simulink model "MSDR_DH_DeplV1sim"  (R2019a)
settings: Solver=ode45  StartTime=0.0  StopTime=simtime  FixedStep=0.1  MaxStep=ts_max  RelTol=rel_tolerance
values from neighbouring files (symbols this model uses):
  a_f = 1E-5*depl_fuel_temp_coef(depl_index)    [MSDR_DH_DeplV1para.m]
  a_g = 1E-5*depl_grap_temp_coef(depl_index)    [MSDR_DH_DeplV1para.m]
  A_s = 1.2245    [MSDR_DH_DeplV1para.m]
  beta = depl_beta(depl_index,:)    [MSDR_DH_DeplV1para.m]
  beta_t = sum(beta)    [MSDR_DH_DeplV1para.m]
  Cp_f = depl_Cp_Fuel_coef*1.355616e-3    [MSDR_DH_DeplV1para.m]
  Cp_p = Cp_s_shx    [MSDR_DH_DeplV1para.m]
  Cp_s = Cp_s*1e-6    (= 3.588208e-09)    [MSDR_DH_DeplV1para.m]
  Cp_sc = 4761.392e-6    (= 0.004761392)    [MSDR_DH_DeplV1para.m]
  Cp_w = 456.056e-6    (= 0.000456056)    [MSDR_DH_DeplV1para.m]
  D_it = 0.0141478    [MSDR_DH_DeplV1para.m]
  D_ot = 0.015875    [MSDR_DH_DeplV1para.m]
  DHRS_TIME_K = 10    [MSDR_DH_DeplV1para.m]
  dHs_dPs = -0.042433622114357    (= -0.0424336221144)    [MSDR_DH_DeplV1para.m]
  Epsilon = 1E-3    (= 0.001)    [MSDR_DH_DeplV1para.m]
  Fiss_factor = 2.464783802008740e-03    (= 0.00246478380201)    [MSDR_DH_DeplV1para.m]
  gamma0 = 9.635981959409105e-01    (= 0.963598195941)    [MSDR_DH_DeplV1para.m]
  gamma1 = 3.560674858154914e-02    (= 0.0356067485815)    [MSDR_DH_DeplV1para.m]
  gamma2 = 7.950554775404400e-04    (= 0.00079505547754)    [MSDR_DH_DeplV1para.m]
  gamma_I = 5.1135e-2    (= 0.051135)    [MSDR_DH_DeplV1para.m]
  gamma_Pm = 1.08E-2    (= 0.0108)    [MSDR_DH_DeplV1para.m]
  gamma_Xe = 1.1628e-2    (= 0.011628)    [MSDR_DH_DeplV1para.m]
  h_pw = h_s_shx    [MSDR_DH_DeplV1para.m]
  h_wb = 13349.334646671E-6    (= 0.0133493346467)    [MSDR_DH_DeplV1para.m]
  h_ws = 5732.378387768E-6    (= 0.00573237838777)    [MSDR_DH_DeplV1para.m]
  h_wsc = 8385.005556375E-6    (= 0.00838500555638)    [MSDR_DH_DeplV1para.m]
  hA_fg = [h_fg*A_fg/2, h_fg*A_fg/2]    [MSDR_DH_DeplV1para.m]
  hA_p_phx1 = h_p_phx*A_p_phx    [MSDR_DH_DeplV1para.m]
  hA_p_phx2 = h_p_phx*A_p_phx    [MSDR_DH_DeplV1para.m]
  hA_p_phx3 = h_p_phx*A_p_phx    [MSDR_DH_DeplV1para.m]
  hA_p_phx4 = h_p_phx*A_p_phx    [MSDR_DH_DeplV1para.m]
  hA_p_phx5 = h_p_phx*A_p_phx    [MSDR_DH_DeplV1para.m]
  hA_p_phx6 = h_p_phx*A_p_phx    [MSDR_DH_DeplV1para.m]
  hA_p_shx1 = h_p_shx*A_p_shx    [MSDR_DH_DeplV1para.m]
  hA_p_shx2 = h_p_shx*A_p_shx    [MSDR_DH_DeplV1para.m]
  hA_p_shx3 = h_p_shx*A_p_shx    [MSDR_DH_DeplV1para.m]
  hA_p_shx4 = h_p_shx*A_p_shx    [MSDR_DH_DeplV1para.m]
  hA_p_shx5 = h_p_shx*A_p_shx    [MSDR_DH_DeplV1para.m]
  hA_p_shx6 = h_p_shx*A_p_shx    [MSDR_DH_DeplV1para.m]
  hA_s_phx1 = h_s_phx*A_s_phx    [MSDR_DH_DeplV1para.m]
  hA_s_phx2 = h_s_phx*A_s_phx    [MSDR_DH_DeplV1para.m]
  hA_s_phx3 = h_s_phx*A_s_phx    [MSDR_DH_DeplV1para.m]
  hA_s_phx4 = h_s_phx*A_s_phx    [MSDR_DH_DeplV1para.m]
  hA_s_phx5 = h_s_phx*A_s_phx    [MSDR_DH_DeplV1para.m]
  hA_s_phx6 = h_s_phx*A_s_phx    [MSDR_DH_DeplV1para.m]
  hA_s_shx1 = h_s_shx*A_s_shx    [MSDR_DH_DeplV1para.m]
  hA_s_shx2 = h_s_shx*A_s_shx    [MSDR_DH_DeplV1para.m]
  hA_s_shx3 = h_s_shx*A_s_shx    [MSDR_DH_DeplV1para.m]
  hA_s_shx4 = h_s_shx*A_s_shx    [MSDR_DH_DeplV1para.m]
  hA_s_shx5 = h_s_shx*A_s_shx    [MSDR_DH_DeplV1para.m]
  hA_s_shx6 = h_s_shx*A_s_shx    [MSDR_DH_DeplV1para.m]
  I_0 = gamma_I*Sig_f_msdr*phi_0/lam_I    [MSDR_DH_DeplV1para.m]
  Ifa = [0.25, 0.25]    [MSDR_DH_DeplV1para.m]
  Ifb = [0.25, 0.25]    [MSDR_DH_DeplV1para.m]
  Ig = [0.5, 0.5]    [MSDR_DH_DeplV1para.m]
  K_1 = 11.632248097704855    (= 11.6322480977)    [MSDR_DH_DeplV1para.m]
  K_4 = b(1)    [MSDR_DH_DeplV1para.m]
  K_5 = a(1)    [MSDR_DH_DeplV1para.m]
  K_b = 12.834854076292217    (= 12.8348540763)    [MSDR_DH_DeplV1para.m]
  K_pump = 1/5    (= 0.2)    [MSDR_DH_DeplV1para.m]
  K_sc = -17.615718797133468    (= -17.6157187971)    [MSDR_DH_DeplV1para.m]
  ka = [0.235, 0.235]    [MSDR_DH_DeplV1para.m]
  kb = [0.235, 0.235]    [MSDR_DH_DeplV1para.m]
  kga = [0.015, 0.015]    [MSDR_DH_DeplV1para.m]
  kgb = [0.015, 0.015]    [MSDR_DH_DeplV1para.m]
  L = 8.5344    [MSDR_DH_DeplV1para.m]
  L_b = 2.3645    [MSDR_DH_DeplV1para.m]
  L_s = 4.723    [MSDR_DH_DeplV1para.m]
  Lam = depl_Lam(depl_index)    [MSDR_DH_DeplV1para.m]
  lam = [1.240E-02, 3.05E-02, 1.11E-01, 3.01E-01, 1.140E+00, 3.014E+00]    [MSDR_DH_DeplV1para.m]
  lam_bubl = 2.0e-2    (= 0.02)    [MSDR_DH_DeplV1para.m]
  lam_I = 2.875e-5    (= 2.875e-05)    [MSDR_DH_DeplV1para.m]
  lam_Pm = log(2)/(2.21*24*3600)    [MSDR_DH_DeplV1para.m]
  lam_Xe = 2.0916e-5    (= 2.0916e-05)    [MSDR_DH_DeplV1para.m]
  lambda0 = 0.0945298    [MSDR_DH_DeplV1para.m]
  lambda1 = 0.00441957    [MSDR_DH_DeplV1para.m]
  lambda2 = 8.60979e-05    [MSDR_DH_DeplV1para.m]
  m_3m = W_3*2    (= 8618.207327)    [MSDR_DH_DeplV1para.m]
  m_f_t = total_mp_phx + core_fm + mp_phxm*3 + m_fm    [MSDR_DH_DeplV1para.m]
  m_fm = W_f*1    (= 4989.48)    [MSDR_DH_DeplV1para.m]
  M_stm = 0.018    [MSDR_DH_DeplV1para.m]
  mcp_fa = mfa*Cp_f    [MSDR_DH_DeplV1para.m]
  mcp_fb = mfb*Cp_f    [MSDR_DH_DeplV1para.m]
  mcp_g = mg*Cp_g    [MSDR_DH_DeplV1para.m]
  mcp_p_phx1 = Cp_p_phx*mp_phx1    [MSDR_DH_DeplV1para.m]
  mcp_p_phx2 = Cp_p_phx*mp_phx2    [MSDR_DH_DeplV1para.m]
  mcp_p_phx3 = Cp_p_phx*mp_phx3    [MSDR_DH_DeplV1para.m]
  mcp_p_phx4 = Cp_p_phx*mp_phx4    [MSDR_DH_DeplV1para.m]
  mcp_p_phx5 = Cp_p_phx*mp_phx5    [MSDR_DH_DeplV1para.m]
  mcp_p_phx6 = Cp_p_phx*mp_phx6    [MSDR_DH_DeplV1para.m]
  mcp_p_shx1 = Cp_p_shx*mp_shx1    [MSDR_DH_DeplV1para.m]
  mcp_p_shx2 = Cp_p_shx*mp_shx2    [MSDR_DH_DeplV1para.m]
  mcp_p_shx3 = Cp_p_shx*mp_shx3    [MSDR_DH_DeplV1para.m]
  mcp_p_shx4 = Cp_p_shx*mp_shx4    [MSDR_DH_DeplV1para.m]
  mcp_p_shx5 = Cp_p_shx*mp_shx5    [MSDR_DH_DeplV1para.m]
  mcp_p_shx6 = Cp_p_shx*mp_shx6    [MSDR_DH_DeplV1para.m]
  mcp_s_phx1 = Cp_s_phx*ms_phx1    [MSDR_DH_DeplV1para.m]
  mcp_s_phx2 = Cp_s_phx*ms_phx2    [MSDR_DH_DeplV1para.m]
  mcp_s_phx3 = Cp_s_phx*ms_phx3    [MSDR_DH_DeplV1para.m]
  mcp_s_phx4 = Cp_s_phx*ms_phx4    [MSDR_DH_DeplV1para.m]
  mcp_s_phx5 = Cp_s_phx*ms_phx5    [MSDR_DH_DeplV1para.m]
  mcp_s_phx6 = Cp_s_phx*ms_phx6    [MSDR_DH_DeplV1para.m]
  mcp_s_shx1 = Cp_s_shx*ms_shx1    [MSDR_DH_DeplV1para.m]
  mcp_s_shx2 = Cp_s_shx*ms_shx1    [MSDR_DH_DeplV1para.m]
  mcp_s_shx3 = Cp_s_shx*ms_shx1    [MSDR_DH_DeplV1para.m]
  mcp_s_shx4 = Cp_s_shx*ms_shx1    [MSDR_DH_DeplV1para.m]
  mcp_s_shx5 = Cp_s_shx*ms_shx1    [MSDR_DH_DeplV1para.m]
  mcp_s_shx6 = Cp_s_shx*ms_shx1    [MSDR_DH_DeplV1para.m]
  mcp_t_phx1 = Cp_t_phx*mt_phx1    [MSDR_DH_DeplV1para.m]
  mcp_t_phx2 = Cp_t_phx*mt_phx2    [MSDR_DH_DeplV1para.m]
  mcp_t_phx3 = Cp_t_phx*mt_phx3    [MSDR_DH_DeplV1para.m]
  mcp_t_phx4 = Cp_t_phx*mt_phx4    [MSDR_DH_DeplV1para.m]
  mcp_t_phx5 = Cp_t_phx*mt_phx5    [MSDR_DH_DeplV1para.m]
  mcp_t_phx6 = Cp_t_phx*mt_phx6    [MSDR_DH_DeplV1para.m]
  mcp_t_shx1 = Cp_t_phx*mt_shx1    [MSDR_DH_DeplV1para.m]
  mcp_t_shx2 = Cp_t_phx*mt_shx2    [MSDR_DH_DeplV1para.m]
  mcp_t_shx3 = Cp_t_phx*mt_shx3    [MSDR_DH_DeplV1para.m]
  mcp_t_shx4 = Cp_t_phx*mt_shx4    [MSDR_DH_DeplV1para.m]
  mcp_t_shx5 = Cp_t_phx*mt_shx5    [MSDR_DH_DeplV1para.m]
  mcp_t_shx6 = Cp_t_phx*mt_shx6    [MSDR_DH_DeplV1para.m]
  ... (+159 more)
undefined symbols (not defined in the file or in its folder): C0, DHRS_MODE, DHRS_Power, DHRS_time, ln, P, Trip_P1_pump, Trip_P2_pump, Trip_P3_pump, Trip_S1_pump, Trip_S2_pump, Trip_S3_pump, Trip_T1_pump, Trip_T2_pump, Trip_T3_pump, Trip_UHX
libraries: simulink x2
(part 2 of 4)

== system MSDR_DH_DeplV1sim/SECONDARY SIDE/OTSG + BALANCE OF PLANT ==
  HITEC_INLET : Inport
  POWER LEVEL : Inport  Port=2
  HITEC_FLOW_FRAC : Inport  Port=3
  HITEC_HTC_FRAC : Inport  Port=4
  Clock : Clock
  Clock1 : Clock
  Constant1 : Constant  Value=0
  Constant12 : Constant  Value=T_fw
  Constant13 : Constant  Value=W_p0
  Constant2 : Constant
  Constant4 : Constant  Value=12.5
  Display{12,14..15,47} (4 alike) : Display
  ONCE-THROUGH STEAM GENERATOR : Subsystem
  Product : Product
  SHX TO PHX DELAY1 : VariableTransportDelay  MaximumDelay=1000000000000  InitialOutput=T0_s_shx5(4)
  Switch : Switch  Criteria=u2 > Threshold  Threshold=Trip_UHX
  Switch1 : Switch  Threshold=Trip_UHX
  VAR DELAY FUNC3 : Fcn  Expr=tau_ostg_shx/u
  HITEC_OUTLET : Outport
  wires:
  ONCE-THROUGH STEAM GENERATOR/4(STEAM FLOW RATE) -> [steam_flow_OTSG], Display15/1
  ONCE-THROUGH STEAM GENERATOR/2(HITEC OUTLET TEMPERATURE) -> Display47/1, Switch/3
  ONCE-THROUGH STEAM GENERATOR/1(STEAM TEMPERATURE) -> Display12/1, [T_steam_OTSG]
  ONCE-THROUGH STEAM GENERATOR/3(STEAM PRESSURE) -> [P_steam_OTSG], Display14/1
  HITEC_INLET/1 -> ONCE-THROUGH STEAM GENERATOR/1(HITEC INLET TEMPERATURE), [HITEC_IN_TEMP]
  Constant4/1 -> ONCE-THROUGH STEAM GENERATOR/6(PRESSURE SET POINT)
  Constant12/1 -> ONCE-THROUGH STEAM GENERATOR/2(FEEDWATER INLET TEMPERATURE)
  HITEC_HTC_FRAC/1 -> ONCE-THROUGH STEAM GENERATOR/4(HITEC HEAT TRANSFER FRAC)
  Constant13/1 -> Product/2
  HITEC_FLOW_FRAC/1 -> Product/1, [HITEC_FLOW_FRAC]
  Product/1 -> ONCE-THROUGH STEAM GENERATOR/3(HITEC FLOW RATE)
  Switch/1 -> HITEC_OUTLET/1
  Clock/1 -> Switch/2
  [HITEC_FLOW_FRAC] -> VAR DELAY FUNC3/1
  [HITEC_IN_TEMP] -> SHX TO PHX DELAY1/1
  VAR DELAY FUNC3/1 -> SHX TO PHX DELAY1/2
  SHX TO PHX DELAY1/1 -> Switch/1
  Clock1/1 -> Switch1/2
  Constant1/1 -> Switch1/1
  POWER LEVEL/1 -> ONCE-THROUGH STEAM GENERATOR/5(POWER)
  Switch1/1 -> ONCE-THROUGH STEAM GENERATOR/Enable
  Constant2/1 -> Switch1/3

== system MSDR_DH_DeplV1sim/SECONDARY SIDE/Variant Subsystem ==
  HITEC_INLET : Inport
  POWER LEVEL : Inport  Port=2
  HITEC_FLOW_FRAC : Inport  Port=3
  HITEC_HTC_FRAC : Inport  Port=4
  OTSG : Subsystem  VariantControl=OTSG
  UHX : Subsystem  VariantControl=UHX
  HITEC_OUTLET : Outport

== system MSDR_DH_DeplV1sim/HEAT EXCHANGERS/HEAT EXCHANGER LOOP 1/PHX PRIM MIXING ==
  Tp_phx1 : Inport
  Tp_phx2 : Inport  Port=2
  p_flow_frac : Inport  Port=3
  Decay Heat : Inport  Port=4
  Fcn : Fcn  Expr=u[3]*Wp_phx1/mp_phxm*(u[1]-u[4]) + u[3]*Wp_phx2/mp_phxm*(u[2]-u[4]) + u(5)*P*mp_phxm/(m_f_t*mp_phxm*Cp_f)
  Integrator : Integrator  InitialCondition=Tf_in
  Mux : Mux  Inputs=5
  Tp_phx_mix : Outport
  wires:
  Tp_phx1/1 -> Mux/1
  Tp_phx2/1 -> Mux/2
  Mux/1 -> Fcn/1
  p_flow_frac/1 -> Mux/3
  Fcn/1 -> Integrator/1
  Integrator/1 -> Mux/4, Tp_phx_mix/1
  Decay Heat/1 -> Mux/5

== system MSDR_DH_DeplV1sim/HEAT EXCHANGERS/HEAT EXCHANGER LOOP 1/PHX SEC MIXING ==
  Ts_phx1 : Inport
  Ts_phx2 : Inport  Port=2
  s_flow_frac : Inport  Port=3
  Fcn : Fcn  Expr=u[3]*Ws_phx1/ms_phxm*(u[1]-u[4]) + u[3]*Ws_phx2/ms_phxm*(u[2]-u[4])
  Integrator : Integrator  InitialCondition=T0_s_phx1(4)
  Mux : Mux
  Ts_phx_mix : Outport
  wires:
  Ts_phx1/1 -> Mux/1
  Ts_phx2/1 -> Mux/2
  Mux/1 -> Fcn/1
  s_flow_frac/1 -> Mux/3
  Fcn/1 -> Integrator/1
  Integrator/1 -> Ts_phx_mix/1, Mux/4

== system MSDR_DH_DeplV1sim/HEAT EXCHANGERS/HEAT EXCHANGER LOOP 1/PHX//SHX PUMP ==
  Clock1 : Clock
  Fcn1 : Fcn  Expr=(1-therm_conv)*exp(-K_pump*(u))+therm_conv
  H.T.C. as f(flow_fraction) : Fcn  Expr=0.8215*u^6-4.108*u^5+7.848*u^4-7.165*u^3+3.004*u^2+0.5903*u+0.008537
  Pump Trip Time : TransportDelay  DelayTime=Trip_S1_pump  BufferSize=4096
  FLOW FRACTION : Outport
  HEAT TRANSFER FRACTION : Outport  Port=2
  wires:
  H.T.C. as f(flow_fraction)/1 -> HEAT TRANSFER FRACTION/1
  Clock1/1 -> Pump Trip Time/1
  Pump Trip Time/1 -> Fcn1/1
  Fcn1/1 -> FLOW FRACTION/1, H.T.C. as f(flow_fraction)/1

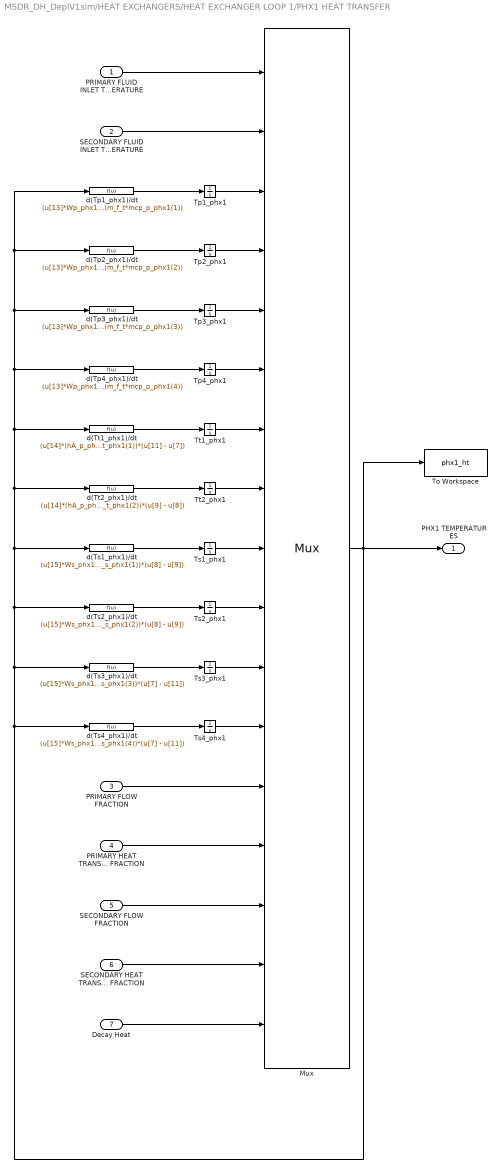
== system MSDR_DH_DeplV1sim/HEAT EXCHANGERS/HEAT EXCHANGER LOOP 1/PHX1 HEAT TRANSFER ==
  PRIMARY FLUID INLET TEMPERATURE : Inport
  SECONDARY FLUID INLET TEMPERATURE : Inport  Port=2
  PRIMARY FLOW FRACTION : Inport  Port=3
  PRIMARY HEAT TRANSFER FRACTION : Inport  Port=4
  SECONDARY FLOW FRACTION : Inport  Port=5
  SECONDARY HEAT TRANSFER FRACTION : Inport  Port=6
  Decay Heat : Inport  Port=7
  Mux : Mux  Inputs=17
      settings: DisplayOption=signals
  To Workspace : ToWorkspace  VariableName=phx1_ht  SampleTime=-1
  Tp1_phx1 : Integrator  InitialCondition=T0_p_phx1(1)
  Tp2_phx1 : Integrator  InitialCondition=T0_p_phx1(2)
  "Tp3_phx1 " : Integrator  InitialCondition=T0_p_phx1(3)
  Tp4_phx1 : Integrator  InitialCondition=T0_p_phx1(4)
  Ts1_phx1 : Integrator  InitialCondition=T0_s_phx1(1)
  Ts2_phx1 : Integrator  InitialCondition=T0_s_phx1(2)
  Ts3_phx1 : Integrator  InitialCondition=T0_s_phx1(3)
  Ts4_phx1 : Integrator  InitialCondition=T0_s_phx1(4)
  Tt1_phx1 : Integrator  InitialCondition=T0_t_phx1(1)
  Tt2_phx1 : Integrator  InitialCondition=T0_t_phx1(2)
  d(Tp1_phx1)/dt : Fcn  Expr=(u[13]*Wp_phx1/mp_phx1(1))*(u[1] - u[3]) + (u[14]*hA_p_phx1(1)/mcp_p_phx1(1))*(u[7] - u[3]) + u(17)*P*mp_phx1(1)/(m_f_t*mcp_p_phx1(1))
  d(Tp2_phx1)/dt : Fcn  Expr=(u[13]*Wp_phx1/mp_phx1(2))*(u[3] - u[4]) + (u[14]*hA_p_phx1(2)/mcp_p_phx1(2))*(u[7] - u[3]) + u(17)*P*mp_phx1(2)/(m_f_t*mcp_p_phx1(2))
  d(Tp3_phx1)/dt : Fcn  Expr=(u[13]*Wp_phx1/mp_phx1(3))*(u[4] - u[5]) + (u[14]*hA_p_phx1(3)/mcp_p_phx1(3))*(u[8] - u[5]) + u(17)*P*mp_phx1(3)/(m_f_t*mcp_p_phx1(3))
  d(Tp4_phx1)/dt : Fcn  Expr=(u[13]*Wp_phx1/mp_phx1(4))*(u[5] - u[6]) + (u[14]*hA_p_phx1(4)/mcp_p_phx1(4))*(u[8] - u[5]) + u(17)*P*mp_phx1(4)/(m_f_t*mcp_p_phx1(4))
  d(Ts1_phx1)/dt : Fcn  Expr=(u[15]*Ws_phx1/ms_phx1(1))*(u[2] - u[9]) + (u[16]*hA_s_phx1(1)/mcp_s_phx1(1))*(u[8] - u[9])
  d(Ts2_phx1)/dt : Fcn  Expr=(u[15]*Ws_phx1/ms_phx1(2))*(u[9] - u[10]) + (u[16]*hA_s_phx1(2)/mcp_s_phx1(2))*(u[8] - u[9])
  d(Ts3_phx1)/dt : Fcn  Expr=(u[15]*Ws_phx1/ms_phx1(3))*(u[10] - u[11]) + (u[16]*hA_s_phx1(3)/mcp_s_phx1(3))*(u[7] - u[11])
  d(Ts4_phx1)/dt : Fcn  Expr=(u[15]*Ws_phx1/ms_phx1(4))*(u[11] - u[12]) + (u[16]*hA_s_phx1(4)/mcp_s_phx1(4))*(u[7] - u[11])
  d(Tt1_phx1)/dt : Fcn  Expr=(u[14]*(hA_p_phx1(1) + hA_p_phx1(2))/mcp_t_phx1(1))*(u[3] - u[7]) + (u[16]*(hA_s_phx1(1) + hA_s_phx1(2))/mcp_t_phx1(1))*(u[11] - u[7])
  d(Tt2_phx1)/dt : Fcn  Expr=(u[14]*(hA_p_phx1(3) + hA_p_phx1(4))/mcp_t_phx1(2))*(u[5] - u[8]) + (u[16]*(hA_s_phx1(3) + hA_s_phx1(4))/mcp_t_phx1(2))*(u[9] - u[8])
  PHX1 TEMPERATURES : Outport
  wires:
  Ts1_phx1/1 -> Mux/9
  Ts2_phx1/1 -> Mux/10
  d(Ts2_phx1)/dt/1 -> Ts2_phx1/1
  d(Tp4_phx1)/dt/1 -> Tp4_phx1/1
  Tt1_phx1/1 -> Mux/7
  d(Tp2_phx1)/dt/1 -> Tp2_phx1/1
  Tp4_phx1/1 -> Mux/6
  d(Tt2_phx1)/dt/1 -> Tt2_phx1/1
  SECONDARY FLUID INLET TEMPERATURE/1 -> Mux/2
  Tt2_phx1/1 -> Mux/8
  Mux/1 -> To Workspace/1, PHX1 TEMPERATURES/1, d(Ts4_phx1)/dt/1, d(Ts3_phx1)/dt/1, d(Ts1_phx1)/dt/1, d(Tt2_phx1)/dt/1, d(Tt1_phx1)/dt/1, d(Tp4_phx1)/dt/1, d(Tp3_phx1)/dt/1, d(Tp2_phx1)/dt/1, d(Tp1_phx1)/dt/1, d(Ts2_phx1)/dt/1
  d(Tp1_phx1)/dt/1 -> Tp1_phx1/1
  d(Ts4_phx1)/dt/1 -> Ts4_phx1/1
  Tp1_phx1/1 -> Mux/3
  d(Ts1_phx1)/dt/1 -> Ts1_phx1/1
  d(Ts3_phx1)/dt/1 -> Ts3_phx1/1
  Ts3_phx1/1 -> Mux/11
  Ts4_phx1/1 -> Mux/12
  "Tp3_phx1 "/1 -> Mux/5
  d(Tp3_phx1)/dt/1 -> "Tp3_phx1 "/1
  Tp2_phx1/1 -> Mux/4
  d(Tt1_phx1)/dt/1 -> Tt1_phx1/1
  PRIMARY FLUID INLET TEMPERATURE/1 -> Mux/1
  PRIMARY FLOW FRACTION/1 -> Mux/13
  PRIMARY HEAT TRANSFER FRACTION/1 -> Mux/14
  SECONDARY HEAT TRANSFER FRACTION/1 -> Mux/16
  SECONDARY FLOW FRACTION/1 -> Mux/15
  Decay Heat/1 -> Mux/17

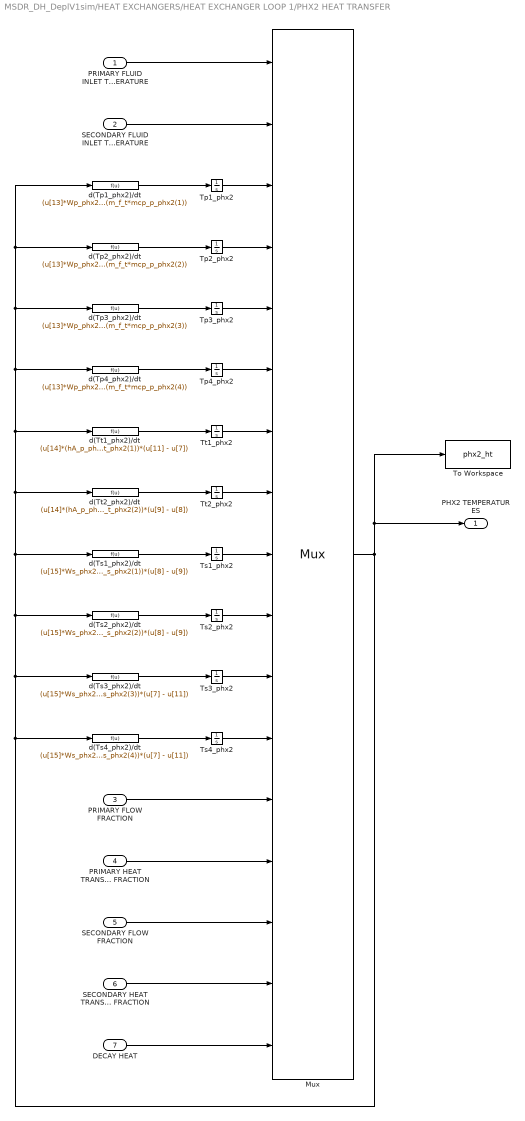
== system MSDR_DH_DeplV1sim/HEAT EXCHANGERS/HEAT EXCHANGER LOOP 1/PHX2 HEAT TRANSFER ==
  PRIMARY FLUID INLET TEMPERATURE : Inport
  SECONDARY FLUID INLET TEMPERATURE : Inport  Port=2
  PRIMARY FLOW FRACTION : Inport  Port=3
  PRIMARY HEAT TRANSFER FRACTION : Inport  Port=4
  SECONDARY FLOW FRACTION : Inport  Port=5
  SECONDARY HEAT TRANSFER FRACTION : Inport  Port=6
  DECAY HEAT : Inport  Port=7
  Mux : Mux  Inputs=17
      settings: DisplayOption=signals
  To Workspace : ToWorkspace  VariableName=phx2_ht  SampleTime=-1
  Tp1_phx2 : Integrator  InitialCondition=T0_p_phx2(1)
  Tp2_phx2 : Integrator  InitialCondition=T0_p_phx1(2)
  "Tp3_phx2 " : Integrator  InitialCondition=T0_p_phx2(3)
  Tp4_phx2 : Integrator  InitialCondition=T0_p_phx2(4)
  Ts1_phx2 : Integrator  InitialCondition=T0_s_phx2(1)
  Ts2_phx2 : Integrator  InitialCondition=T0_s_phx2(2)
  Ts3_phx2 : Integrator  InitialCondition=T0_s_phx2(3)
  Ts4_phx2 : Integrator  InitialCondition=T0_s_phx2(4)
  Tt1_phx2 : Integrator  InitialCondition=T0_t_phx2(1)
  Tt2_phx2 : Integrator  InitialCondition=T0_t_phx2(2)
  d(Tp1_phx2)/dt : Fcn  Expr=(u[13]*Wp_phx2/mp_phx2(1))*(u[1] - u[3]) + (u[14]*hA_p_phx2(1)/mcp_p_phx2(1))*(u[7] - u[3]) + u(17)*P*mp_phx2(1)/(m_f_t*mcp_p_phx2(1))
  d(Tp2_phx2)/dt : Fcn  Expr=(u[13]*Wp_phx2/mp_phx2(2))*(u[3] - u[4]) + (u[14]*hA_p_phx2(2)/mcp_p_phx2(2))*(u[7] - u[3]) + u(17)*P*mp_phx2(2)/(m_f_t*mcp_p_phx2(2))
  d(Tp3_phx2)/dt : Fcn  Expr=(u[13]*Wp_phx2/mp_phx2(3))*(u[4] - u[5]) + (u[14]*hA_p_phx2(3)/mcp_p_phx2(3))*(u[8] - u[5]) + u(17)*P*mp_phx2(3)/(m_f_t*mcp_p_phx2(3))
  d(Tp4_phx2)/dt : Fcn  Expr=(u[13]*Wp_phx2/mp_phx2(4))*(u[5] - u[6]) + (u[14]*hA_p_phx2(4)/mcp_p_phx2(4))*(u[8] - u[5]) + u(17)*P*mp_phx2(4)/(m_f_t*mcp_p_phx2(4))
  d(Ts1_phx2)/dt : Fcn  Expr=(u[15]*Ws_phx2/ms_phx2(1))*(u[2] - u[9]) + (u[16]*hA_s_phx2(1)/mcp_s_phx2(1))*(u[8] - u[9])
  d(Ts2_phx2)/dt : Fcn  Expr=(u[15]*Ws_phx2/ms_phx2(2))*(u[9] - u[10]) + (u[16]*hA_s_phx2(2)/mcp_s_phx2(2))*(u[8] - u[9])
  d(Ts3_phx2)/dt : Fcn  Expr=(u[15]*Ws_phx2/ms_phx2(3))*(u[10] - u[11]) + (u[16]*hA_s_phx2(3)/mcp_s_phx2(3))*(u[7] - u[11])
  d(Ts4_phx2)/dt : Fcn  Expr=(u[15]*Ws_phx2/ms_phx2(4))*(u[11] - u[12]) + (u[16]*hA_s_phx2(4)/mcp_s_phx2(4))*(u[7] - u[11])
  d(Tt1_phx2)/dt : Fcn  Expr=(u[14]*(hA_p_phx2(1) + hA_p_phx2(2))/mcp_t_phx2(1))*(u[3] - u[7]) + (u[16]*(hA_s_phx2(1) + hA_s_phx2(2))/mcp_t_phx2(1))*(u[11] - u[7])
  d(Tt2_phx2)/dt : Fcn  Expr=(u[14]*(hA_p_phx2(3) + hA_p_phx2(4))/mcp_t_phx2(2))*(u[5] - u[8]) + (u[16]*(hA_s_phx2(3) + hA_s_phx2(4))/mcp_t_phx2(2))*(u[9] - u[8])
  PHX2 TEMPERATURES : Outport
  wires:
  Ts1_phx2/1 -> Mux/9
  Ts2_phx2/1 -> Mux/10
  d(Ts2_phx2)/dt/1 -> Ts2_phx2/1
  d(Tp4_phx2)/dt/1 -> Tp4_phx2/1
  Tt1_phx2/1 -> Mux/7
  d(Tp2_phx2)/dt/1 -> Tp2_phx2/1
  Tp4_phx2/1 -> Mux/6
  d(Tt2_phx2)/dt/1 -> Tt2_phx2/1
  SECONDARY FLUID INLET TEMPERATURE/1 -> Mux/2
  Tt2_phx2/1 -> Mux/8
  Mux/1 -> To Workspace/1, PHX2 TEMPERATURES/1, d(Ts4_phx2)/dt/1, d(Ts3_phx2)/dt/1, d(Ts1_phx2)/dt/1, d(Tt2_phx2)/dt/1, d(Tt1_phx2)/dt/1, d(Tp4_phx2)/dt/1, d(Tp3_phx2)/dt/1, d(Tp2_phx2)/dt/1, d(Tp1_phx2)/dt/1, d(Ts2_phx2)/dt/1
  d(Tp1_phx2)/dt/1 -> Tp1_phx2/1
  d(Ts4_phx2)/dt/1 -> Ts4_phx2/1
  Tp1_phx2/1 -> Mux/3
  d(Ts1_phx2)/dt/1 -> Ts1_phx2/1
  d(Ts3_phx2)/dt/1 -> Ts3_phx2/1
  Ts3_phx2/1 -> Mux/11
  Ts4_phx2/1 -> Mux/12
  "Tp3_phx2 "/1 -> Mux/5
  d(Tp3_phx2)/dt/1 -> "Tp3_phx2 "/1
  Tp2_phx2/1 -> Mux/4
  d(Tt1_phx2)/dt/1 -> Tt1_phx2/1
  PRIMARY FLUID INLET TEMPERATURE/1 -> Mux/1
  PRIMARY FLOW FRACTION/1 -> Mux/13
  PRIMARY HEAT TRANSFER FRACTION/1 -> Mux/14
  SECONDARY FLOW FRACTION/1 -> Mux/15
  SECONDARY HEAT TRANSFER FRACTION/1 -> Mux/16
  DECAY HEAT/1 -> Mux/17

== system MSDR_DH_DeplV1sim/HEAT EXCHANGERS/HEAT EXCHANGER LOOP 1/SHX PRIM MIXING ==
  Tp_shx1 : Inport
  Tp_shx2 : Inport  Port=2
  p_flow_frac : Inport  Port=3
  Fcn : Fcn  Expr=u[3]*Wp_shx1/mp_shxm*(u[1]-u[4]) + u[3]*Wp_shx2/mp_shxm*(u[2]-u[4])
  Integrator : Integrator  InitialCondition=T0_p_shx1(4)
  Mux : Mux
  Tp_shx_mix : Outport
  wires:
  Tp_shx1/1 -> Mux/1
  Tp_shx2/1 -> Mux/2
  Mux/1 -> Fcn/1
  p_flow_frac/1 -> Mux/3
  Fcn/1 -> Integrator/1
  Integrator/1 -> Tp_shx_mix/1, Mux/4

== system MSDR_DH_DeplV1sim/HEAT EXCHANGERS/HEAT EXCHANGER LOOP 1/SHX SEC MIXING ==
  Ts_shx1 : Inport
  Ts_shx2 : Inport  Port=2
  s_flow_frac : Inport  Port=3
  Fcn : Fcn  Expr=u[3]*Ws_shx1/ms_shxm*(u[1]-u[4]) + u[3]*Ws_shx2/ms_shxm*(u[2]-u[4])
  Integrator : Integrator  InitialCondition=T0_s_shx1(4)
  Mux : Mux
  Ts_shx_mix : Outport
  wires:
  Ts_shx1/1 -> Mux/1
  Ts_shx2/1 -> Mux/2
  Mux/1 -> Fcn/1
  s_flow_frac/1 -> Mux/3
  Fcn/1 -> Integrator/1
  Integrator/1 -> Ts_shx_mix/1, Mux/4

== system MSDR_DH_DeplV1sim/HEAT EXCHANGERS/HEAT EXCHANGER LOOP 1/SHX//THX PUMP ==
  Clock1 : Clock
  Fcn1 : Fcn  Expr=(1-therm_conv)*exp(-K_pump*(u))+therm_conv
  H.T.C. as f(flow_fraction) : Fcn  Expr=0.8215*u^6-4.108*u^5+7.848*u^4-7.165*u^3+3.004*u^2+0.5903*u+0.008537
  Pump Trip Time : TransportDelay  DelayTime=Trip_T1_pump  BufferSize=4096
  FLOW FRACTION : Outport
  HEAT TRANSFER FRACTION : Outport  Port=2
  wires:
  H.T.C. as f(flow_fraction)/1 -> HEAT TRANSFER FRACTION/1
  Clock1/1 -> Pump Trip Time/1
  Pump Trip Time/1 -> Fcn1/1
  Fcn1/1 -> FLOW FRACTION/1, H.T.C. as f(flow_fraction)/1

== system MSDR_DH_DeplV1sim/HEAT EXCHANGERS/HEAT EXCHANGER LOOP 1/SHX1 HEAT TRANSFER ==
  PRIMARY FLUID INLET TEMPERATURE : Inport
  SECONDARY FLUID INLET TEMPERATURE : Inport  Port=2
  PRIMARY FLOW FRACTION : Inport  Port=3
  PRIMARY HEAT TRANSFER FRACTION : Inport  Port=4
  SECONDARY FLOW FRACTION : Inport  Port=5
  SECONDARY HEAT TRANSFER FRACTION : Inport  Port=6
  Mux : Mux  Inputs=16
      settings: DisplayOption=signals
  To Workspace : ToWorkspace  VariableName=shx1_ht  SampleTime=-1
  Tp1_shx1 : Integrator  InitialCondition=T0_p_shx1(1)
  Tp2_shx1 : Integrator  InitialCondition=T0_p_shx1(2)
  "Tp3_shx1 " : Integrator  InitialCondition=T0_p_shx1(3)
  Tp4_shx1 : Integrator  InitialCondition=T0_p_shx1(4)
  Ts1_shx1 : Integrator  InitialCondition=T0_s_shx1(1)
  Ts2_shx1 : Integrator  InitialCondition=T0_s_shx1(2)
  Ts3_shx1 : Integrator  InitialCondition=T0_s_shx1(3)
  Ts4_shx1 : Integrator  InitialCondition=T0_s_shx1(4)
  Tt1_shx1 : Integrator  InitialCondition=T0_t_shx1(1)
  Tt2_shx1 : Integrator  InitialCondition=T0_t_shx1(2)
  d(Tp1_shx1)/dt : Fcn  Expr=(u[13]*Wp_shx1/mp_shx1(1))*(u[1] - u[3]) + (u[14]*hA_p_shx1(1)/mcp_p_shx1(1))*(u[7] - u[3])
  d(Tp2_shx1)/dt : Fcn  Expr=(u[13]*Wp_shx1/mp_shx1(2))*(u[3] - u[4]) + (u[14]*hA_p_shx1(2)/mcp_p_shx1(2))*(u[7] - u[3])
  d(Tp3_shx1)/dt : Fcn  Expr=(u[13]*Wp_shx1/mp_shx1(3))*(u[4] - u[5]) + (u[14]*hA_p_shx1(3)/mcp_p_shx1(3))*(u[8] - u[5])
  d(Tp4_shx1)/dt : Fcn  Expr=(u[13]*Wp_shx1/mp_shx1(4))*(u[5] - u[6]) + (u[14]*hA_p_shx1(4)/mcp_p_shx1(4))*(u[8] - u[5])
  d(Ts1_shx1)/dt : Fcn  Expr=(u[15]*Ws_shx1/ms_shx1(1))*(u[2] - u[9]) + (u[16]*hA_s_shx1(1)/mcp_s_shx1(1))*(u[8] - u[9])
  d(Ts2_shx1)/dt : Fcn  Expr=(u[15]*Ws_shx1/ms_shx1(2))*(u[9] - u[10]) + (u[16]*hA_s_shx1(2)/mcp_s_shx1(2))*(u[8] - u[9])
  d(Ts3_shx1)/dt : Fcn  Expr=(u[15]*Ws_shx1/ms_shx1(3))*(u[10] - u[11]) + (u[16]*hA_s_shx1(3)/mcp_s_shx1(3))*(u[7] - u[11])
  d(Ts4_shx1)/dt : Fcn  Expr=(u[15]*Ws_shx1/ms_shx1(4))*(u[11] - u[12]) + (u[16]*hA_s_shx1(4)/mcp_s_shx1(4))*(u[7] - u[11])
  d(Tt1_shx1)/dt : Fcn  Expr=(u[14]*(hA_p_shx1(1) + hA_p_shx1(2))/mcp_t_shx1(1))*(u[3] - u[7]) + (u[16]*(hA_s_shx1(1) + hA_s_shx1(2))/mcp_t_shx1(1))*(u[11] - u[7])
  d(Tt2_shx1)/dt : Fcn  Expr=(u[14]*(hA_p_shx1(3) + hA_p_shx1(4))/mcp_t_shx1(2))*(u[5] - u[8]) + (u[16]*(hA_s_shx1(3) + hA_s_shx1(4))/mcp_t_shx1(2))*(u[9] - u[8])
  SHX1 TEMPERATURES : Outport
  wires:
  Ts1_shx1/1 -> Mux/9
  Ts2_shx1/1 -> Mux/10
  d(Ts2_shx1)/dt/1 -> Ts2_shx1/1
  d(Tp4_shx1)/dt/1 -> Tp4_shx1/1
  Tt1_shx1/1 -> Mux/7
  d(Tp2_shx1)/dt/1 -> Tp2_shx1/1
  Tp4_shx1/1 -> Mux/6
  d(Tt2_shx1)/dt/1 -> Tt2_shx1/1
  SECONDARY FLUID INLET TEMPERATURE/1 -> Mux/2
  Tt2_shx1/1 -> Mux/8
  Mux/1 -> To Workspace/1, SHX1 TEMPERATURES/1, d(Ts4_shx1)/dt/1, d(Ts3_shx1)/dt/1, d(Ts2_shx1)/dt/1, d(Ts1_shx1)/dt/1, d(Tt2_shx1)/dt/1, d(Tt1_shx1)/dt/1, d(Tp4_shx1)/dt/1, d(Tp3_shx1)/dt/1, d(Tp2_shx1)/dt/1, d(Tp1_shx1)/dt/1
  d(Tp1_shx1)/dt/1 -> Tp1_shx1/1
  d(Ts4_shx1)/dt/1 -> Ts4_shx1/1
  Tp1_shx1/1 -> Mux/3
  d(Ts1_shx1)/dt/1 -> Ts1_shx1/1
  d(Ts3_shx1)/dt/1 -> Ts3_shx1/1
  Ts3_shx1/1 -> Mux/11
  Ts4_shx1/1 -> Mux/12
  "Tp3_shx1 "/1 -> Mux/5
  d(Tp3_shx1)/dt/1 -> "Tp3_shx1 "/1
  Tp2_shx1/1 -> Mux/4
  d(Tt1_shx1)/dt/1 -> Tt1_shx1/1
  PRIMARY FLUID INLET TEMPERATURE/1 -> Mux/1
  PRIMARY HEAT TRANSFER FRACTION/1 -> Mux/14
  SECONDARY HEAT TRANSFER FRACTION/1 -> Mux/16
  PRIMARY FLOW FRACTION/1 -> Mux/13
  SECONDARY FLOW FRACTION/1 -> Mux/15

== system MSDR_DH_DeplV1sim/HEAT EXCHANGERS/HEAT EXCHANGER LOOP 1/SHX2 HEAT TRANSFER ==
  PRIMARY FLUID INLET TEMPERATURE : Inport
  SECONDARY FLUID INLET TEMPERATURE : Inport  Port=2
  PRIMARY FLOW FRACTION : Inport  Port=3
  PRIMARY HEAT TRANSFER FRACTION : Inport  Port=4
  SECONDARY FLOW FRACTION : Inport  Port=5
  SECONDARY HEAT TRANSFER FRACTION : Inport  Port=6
  Mux : Mux  Inputs=16
      settings: DisplayOption=signals
  To Workspace : ToWorkspace  VariableName=shx2_ht  SampleTime=-1
  Tp1_shx2 : Integrator  InitialCondition=T0_p_shx2(1)
  Tp2_shx2 : Integrator  InitialCondition=T0_p_shx2(2)
  "Tp3_shx2 " : Integrator  InitialCondition=T0_p_shx2(3)
  Tp4_shx2 : Integrator  InitialCondition=T0_p_shx2(4)
  Ts1_shx2 : Integrator  InitialCondition=T0_s_shx2(1)
  Ts2_shx2 : Integrator  InitialCondition=T0_s_shx2(2)
  Ts3_shx2 : Integrator  InitialCondition=T0_s_shx2(3)
  Ts4_shx2 : Integrator  InitialCondition=T0_s_shx2(4)
  Tt1_shx2 : Integrator  InitialCondition=T0_t_shx2(1)
  Tt2_shx2 : Integrator  InitialCondition=T0_t_shx2(2)
  d(Tp1_shx2)/dt : Fcn  Expr=(u[13]*Wp_shx2/mp_shx2(1))*(u[1] - u[3]) + (u[14]*hA_p_shx2(1)/mcp_p_shx2(1))*(u[7] - u[3])
  d(Tp2_shx2)/dt : Fcn  Expr=(u[13]*Wp_shx2/mp_shx2(2))*(u[3] - u[4]) + (u[14]*hA_p_shx2(2)/mcp_p_shx2(2))*(u[7] - u[3])
  d(Tp3_shx2)/dt : Fcn  Expr=(u[13]*Wp_shx2/mp_shx2(3))*(u[4] - u[5]) + (u[14]*hA_p_shx2(3)/mcp_p_shx2(3))*(u[8] - u[5])
  d(Tp4_shx2)/dt : Fcn  Expr=(u[13]*Wp_shx2/mp_shx2(4))*(u[5] - u[6]) + (u[14]*hA_p_shx2(4)/mcp_p_shx2(4))*(u[8] - u[5])
  d(Ts1_shx2)/dt : Fcn  Expr=(u[15]*Ws_shx2/ms_shx2(1))*(u[2] - u[9]) + (u[16]*hA_s_shx2(1)/mcp_s_shx2(1))*(u[8] - u[9])
  d(Ts2_shx2)/dt : Fcn  Expr=(u[15]*Ws_shx2/ms_shx2(2))*(u[9] - u[10]) + (u[16]*hA_s_shx2(2)/mcp_s_shx2(2))*(u[8] - u[9])
  d(Ts3_shx2)/dt : Fcn  Expr=(u[15]*Ws_shx2/ms_shx2(3))*(u[10] - u[11]) + (u[16]*hA_s_shx2(3)/mcp_s_shx2(3))*(u[7] - u[11])
  d(Ts4_shx2)/dt : Fcn  Expr=(u[15]*Ws_shx2/ms_shx2(4))*(u[11] - u[12]) + (u[16]*hA_s_shx2(4)/mcp_s_shx2(4))*(u[7] - u[11])
  d(Tt1_shx2)/dt : Fcn  Expr=(u[14]*(hA_p_shx2(1) + hA_p_shx2(2))/mcp_t_shx2(1))*(u[3] - u[7]) + (u[16]*(hA_s_shx2(1) + hA_s_shx2(2))/mcp_t_shx2(1))*(u[11] - u[7])
  d(Tt2_shx2)/dt : Fcn  Expr=(u[14]*(hA_p_shx2(3) + hA_p_shx2(4))/mcp_t_shx2(2))*(u[5] - u[8]) + (u[16]*(hA_s_shx2(3) + hA_s_shx2(4))/mcp_t_shx2(2))*(u[9] - u[8])
  SHX2 TEMPERATURES : Outport
  wires:
  Ts1_shx2/1 -> Mux/9
  Ts2_shx2/1 -> Mux/10
  d(Ts2_shx2)/dt/1 -> Ts2_shx2/1
  d(Tp4_shx2)/dt/1 -> Tp4_shx2/1
  Tt1_shx2/1 -> Mux/7
  d(Tp2_shx2)/dt/1 -> Tp2_shx2/1
  Tp4_shx2/1 -> Mux/6
  d(Tt2_shx2)/dt/1 -> Tt2_shx2/1
  SECONDARY FLUID INLET TEMPERATURE/1 -> Mux/2
  Tt2_shx2/1 -> Mux/8
  Mux/1 -> To Workspace/1, SHX2 TEMPERATURES/1, d(Ts4_shx2)/dt/1, d(Ts3_shx2)/dt/1, d(Ts2_shx2)/dt/1, d(Ts1_shx2)/dt/1, d(Tt2_shx2)/dt/1, d(Tt1_shx2)/dt/1, d(Tp4_shx2)/dt/1, d(Tp3_shx2)/dt/1, d(Tp2_shx2)/dt/1, d(Tp1_shx2)/dt/1
  d(Tp1_shx2)/dt/1 -> Tp1_shx2/1
  d(Ts4_shx2)/dt/1 -> Ts4_shx2/1
  Tp1_shx2/1 -> Mux/3
  d(Ts1_shx2)/dt/1 -> Ts1_shx2/1
  d(Ts3_shx2)/dt/1 -> Ts3_shx2/1
  Ts3_shx2/1 -> Mux/11
  Ts4_shx2/1 -> Mux/12
  "Tp3_shx2 "/1 -> Mux/5
  d(Tp3_shx2)/dt/1 -> "Tp3_shx2 "/1
  Tp2_shx2/1 -> Mux/4
  d(Tt1_shx2)/dt/1 -> Tt1_shx2/1
  PRIMARY FLUID INLET TEMPERATURE/1 -> Mux/1
  PRIMARY HEAT TRANSFER FRACTION/1 -> Mux/14
  SECONDARY FLOW FRACTION/1 -> Mux/15
  SECONDARY HEAT TRANSFER FRACTION/1 -> Mux/16
  PRIMARY FLOW FRACTION/1 -> Mux/13

== system MSDR_DH_DeplV1sim/HEAT EXCHANGERS/HEAT EXCHANGER LOOP 2/PHX PRIM MIXING ==
  Tp_phx3 : Inport
  Tp_phx4 : Inport  Port=2
  p_flow_frac : Inport  Port=3
  Decay Heat : Inport  Port=4
  Fcn : Fcn  Expr="u[3]*Wp_phx3/mp_phxm*(u[1]-u[4]) + u[3]*Wp_phx4/mp_phxm*(u[2]-u[4])  + u(5)*P*mp_phxm/(m_f_t*mp_phxm*Cp_f)"
  Integrator : Integrator  InitialCondition=Tf_in
  Mux : Mux  Inputs=5
  Tp_phx_mix : Outport
  wires:
  Tp_phx3/1 -> Mux/1
  Tp_phx4/1 -> Mux/2
  Mux/1 -> Fcn/1
  p_flow_frac/1 -> Mux/3
  Fcn/1 -> Integrator/1
  Integrator/1 -> Mux/4, Tp_phx_mix/1
  Decay Heat/1 -> Mux/5

== system MSDR_DH_DeplV1sim/HEAT EXCHANGERS/HEAT EXCHANGER LOOP 2/PHX SEC MIXING ==
  Ts_phx3 : Inport
  Ts_phx4 : Inport  Port=2
  s_flow_frac : Inport  Port=3
  Fcn : Fcn  Expr=u[3]*Ws_phx3/ms_phxm*(u[1]-u[4]) + u[3]*Ws_phx4/ms_phxm*(u[2]-u[4])
  Integrator : Integrator  InitialCondition=T0_s_phx1(4)
  Mux : Mux
  Ts_phx_mix : Outport
  wires:
  Ts_phx3/1 -> Mux/1
  Ts_phx4/1 -> Mux/2
  Mux/1 -> Fcn/1
  s_flow_frac/1 -> Mux/3
  Fcn/1 -> Integrator/1
  Integrator/1 -> Ts_phx_mix/1, Mux/4

== system MSDR_DH_DeplV1sim/HEAT EXCHANGERS/HEAT EXCHANGER LOOP 2/PHX//SHX PUMP ==
  Clock1 : Clock
  Fcn1 : Fcn  Expr=(1-therm_conv)*exp(-K_pump*(u))+therm_conv
  H.T.C. as f(flow_fraction) : Fcn  Expr=0.8215*u^6-4.108*u^5+7.848*u^4-7.165*u^3+3.004*u^2+0.5903*u+0.008537
  Pump Trip Time : TransportDelay  DelayTime=Trip_S2_pump  BufferSize=4096
  FLOW FRACTION : Outport
  HEAT TRANSFER FRACTION : Outport  Port=2
  wires:
  H.T.C. as f(flow_fraction)/1 -> HEAT TRANSFER FRACTION/1
  Clock1/1 -> Pump Trip Time/1
  Pump Trip Time/1 -> Fcn1/1
  Fcn1/1 -> FLOW FRACTION/1, H.T.C. as f(flow_fraction)/1

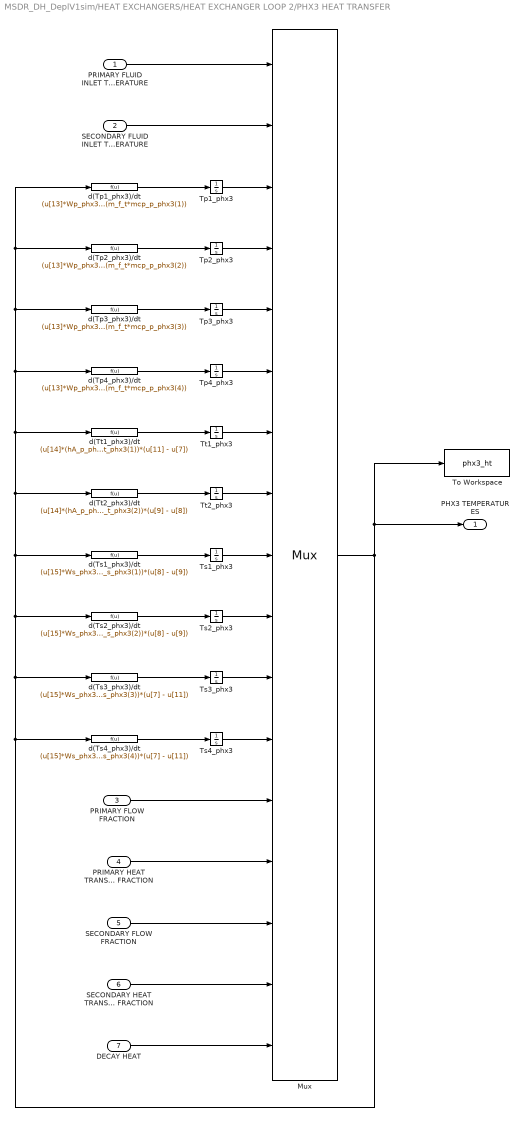
== system MSDR_DH_DeplV1sim/HEAT EXCHANGERS/HEAT EXCHANGER LOOP 2/PHX3 HEAT TRANSFER ==
  PRIMARY FLUID INLET TEMPERATURE : Inport
  SECONDARY FLUID INLET TEMPERATURE : Inport  Port=2
  PRIMARY FLOW FRACTION : Inport  Port=3
  PRIMARY HEAT TRANSFER FRACTION : Inport  Port=4
  SECONDARY FLOW FRACTION : Inport  Port=5
  SECONDARY HEAT TRANSFER FRACTION : Inport  Port=6
  DECAY HEAT : Inport  Port=7
  Mux : Mux  Inputs=17
      settings: DisplayOption=signals
  To Workspace : ToWorkspace  VariableName=phx3_ht  SampleTime=-1
  Tp1_phx3 : Integrator  InitialCondition=T0_p_phx3(1)
  Tp2_phx3 : Integrator  InitialCondition=T0_p_phx3(2)
  "Tp3_phx3 " : Integrator  InitialCondition=T0_p_phx3(3)
  Tp4_phx3 : Integrator  InitialCondition=T0_p_phx3(4)
  Ts1_phx3 : Integrator  InitialCondition=T0_s_phx3(1)
  Ts2_phx3 : Integrator  InitialCondition=T0_s_phx3(2)
  Ts3_phx3 : Integrator  InitialCondition=T0_s_phx3(3)
  Ts4_phx3 : Integrator  InitialCondition=T0_s_phx3(4)
  Tt1_phx3 : Integrator  InitialCondition=T0_t_phx3(1)
  Tt2_phx3 : Integrator  InitialCondition=T0_t_phx3(2)
  d(Tp1_phx3)/dt : Fcn  Expr=(u[13]*Wp_phx3/mp_phx3(1))*(u[1] - u[3]) + (u[14]*hA_p_phx3(1)/mcp_p_phx3(1))*(u[7] - u[3]) + u(17)*P*mp_phx3(1)/(m_f_t*mcp_p_phx3(1))
  d(Tp2_phx3)/dt : Fcn  Expr=(u[13]*Wp_phx3/mp_phx3(2))*(u[3] - u[4]) + (u[14]*hA_p_phx3(2)/mcp_p_phx3(2))*(u[7] - u[3]) + u(17)*P*mp_phx3(2)/(m_f_t*mcp_p_phx3(2))
  d(Tp3_phx3)/dt : Fcn  Expr=(u[13]*Wp_phx3/mp_phx3(3))*(u[4] - u[5]) + (u[14]*hA_p_phx3(3)/mcp_p_phx3(3))*(u[8] - u[5]) + u(17)*P*mp_phx3(3)/(m_f_t*mcp_p_phx3(3))
  d(Tp4_phx3)/dt : Fcn  Expr=(u[13]*Wp_phx3/mp_phx3(4))*(u[5] - u[6]) + (u[14]*hA_p_phx3(4)/mcp_p_phx3(4))*(u[8] - u[5]) + u(17)*P*mp_phx3(4)/(m_f_t*mcp_p_phx3(4))
  d(Ts1_phx3)/dt : Fcn  Expr=(u[15]*Ws_phx3/ms_phx3(1))*(u[2] - u[9]) + (u[16]*hA_s_phx3(1)/mcp_s_phx3(1))*(u[8] - u[9])
  d(Ts2_phx3)/dt : Fcn  Expr=(u[15]*Ws_phx3/ms_phx3(2))*(u[9] - u[10]) + (u[16]*hA_s_phx3(2)/mcp_s_phx3(2))*(u[8] - u[9])
  d(Ts3_phx3)/dt : Fcn  Expr=(u[15]*Ws_phx3/ms_phx3(3))*(u[10] - u[11]) + (u[16]*hA_s_phx3(3)/mcp_s_phx3(3))*(u[7] - u[11])
  d(Ts4_phx3)/dt : Fcn  Expr=(u[15]*Ws_phx3/ms_phx3(4))*(u[11] - u[12]) + (u[16]*hA_s_phx3(4)/mcp_s_phx3(4))*(u[7] - u[11])
  d(Tt1_phx3)/dt : Fcn  Expr=(u[14]*(hA_p_phx3(1) + hA_p_phx3(2))/mcp_t_phx3(1))*(u[3] - u[7]) + (u[16]*(hA_s_phx3(1) + hA_s_phx3(2))/mcp_t_phx3(1))*(u[11] - u[7])
  d(Tt2_phx3)/dt : Fcn  Expr=(u[14]*(hA_p_phx3(3) + hA_p_phx3(4))/mcp_t_phx3(2))*(u[5] - u[8]) + (u[16]*(hA_s_phx3(3) + hA_s_phx3(4))/mcp_t_phx3(2))*(u[9] - u[8])
  PHX3 TEMPERATURES : Outport
  wires:
  Ts1_phx3/1 -> Mux/9
  Ts2_phx3/1 -> Mux/10
  d(Ts2_phx3)/dt/1 -> Ts2_phx3/1
  d(Tp4_phx3)/dt/1 -> Tp4_phx3/1
  Tt1_phx3/1 -> Mux/7
  d(Tp2_phx3)/dt/1 -> Tp2_phx3/1
  Tp4_phx3/1 -> Mux/6
  d(Tt2_phx3)/dt/1 -> Tt2_phx3/1
  SECONDARY FLUID INLET TEMPERATURE/1 -> Mux/2
  Tt2_phx3/1 -> Mux/8
  Mux/1 -> To Workspace/1, PHX3 TEMPERATURES/1, d(Ts4_phx3)/dt/1, d(Ts3_phx3)/dt/1, d(Ts1_phx3)/dt/1, d(Tt2_phx3)/dt/1, d(Tt1_phx3)/dt/1, d(Tp4_phx3)/dt/1, d(Tp3_phx3)/dt/1, d(Tp2_phx3)/dt/1, d(Tp1_phx3)/dt/1, d(Ts2_phx3)/dt/1
  d(Tp1_phx3)/dt/1 -> Tp1_phx3/1
  d(Ts4_phx3)/dt/1 -> Ts4_phx3/1
  Tp1_phx3/1 -> Mux/3
  d(Ts1_phx3)/dt/1 -> Ts1_phx3/1
  d(Ts3_phx3)/dt/1 -> Ts3_phx3/1
  Ts3_phx3/1 -> Mux/11
  Ts4_phx3/1 -> Mux/12
  "Tp3_phx3 "/1 -> Mux/5
  d(Tp3_phx3)/dt/1 -> "Tp3_phx3 "/1
  Tp2_phx3/1 -> Mux/4
  d(Tt1_phx3)/dt/1 -> Tt1_phx3/1
  PRIMARY FLUID INLET TEMPERATURE/1 -> Mux/1
  PRIMARY FLOW FRACTION/1 -> Mux/13
  PRIMARY HEAT TRANSFER FRACTION/1 -> Mux/14
  SECONDARY FLOW FRACTION/1 -> Mux/15
  SECONDARY HEAT TRANSFER FRACTION/1 -> Mux/16
  DECAY HEAT/1 -> Mux/17

== system MSDR_DH_DeplV1sim/HEAT EXCHANGERS/HEAT EXCHANGER LOOP 2/PHX4 HEAT TRANSFER ==
  PRIMARY FLUID INLET TEMPERATURE : Inport
  SECONDARY FLUID INLET TEMPERATURE : Inport  Port=2
  PRIMARY FLOW FRACTION : Inport  Port=3
  PRIMARY HEAT TRANSFER FRACTION : Inport  Port=4
  SECONDARY FLOW FRACTION : Inport  Port=5
  SECONDARY HEAT TRANSFER FRACTION : Inport  Port=6
  DECAY HEAT : Inport  Port=7
  Mux : Mux  Inputs=17
      settings: DisplayOption=signals
  To Workspace : ToWorkspace  VariableName=phx4_ht  SampleTime=-1
  Tp1_phx4 : Integrator  InitialCondition=T0_p_phx4(1)
  Tp2_phx4 : Integrator  InitialCondition=T0_p_phx4(2)
  "Tp3_phx4 " : Integrator  InitialCondition=T0_p_phx4(3)
  Tp4_phx4 : Integrator  InitialCondition=T0_p_phx4(4)
  Ts1_phx4 : Integrator  InitialCondition=T0_s_phx4(1)
  Ts2_phx4 : Integrator  InitialCondition=T0_s_phx4(2)
  Ts3_phx4 : Integrator  InitialCondition=T0_s_phx4(3)
  Ts4_phx4 : Integrator  InitialCondition=T0_s_phx4(4)
  Tt1_phx4 : Integrator  InitialCondition=T0_t_phx4(1)
  Tt2_phx4 : Integrator  InitialCondition=T0_t_phx4(2)
  d(Tp1_phx4)/dt : Fcn  Expr=(u[13]*Wp_phx4/mp_phx4(1))*(u[1] - u[3]) + (u[14]*hA_p_phx4(1)/mcp_p_phx4(1))*(u[7] - u[3]) + u(17)*P*mp_phx4(1)/(m_f_t*mcp_p_phx4(1))
  d(Tp2_phx4)/dt : Fcn  Expr=(u[13]*Wp_phx4/mp_phx4(2))*(u[3] - u[4]) + (u[14]*hA_p_phx4(2)/mcp_p_phx4(2))*(u[7] - u[3]) + u(17)*P*mp_phx4(2)/(m_f_t*mcp_p_phx4(2))
  d(Tp3_phx4)/dt : Fcn  Expr=(u[13]*Wp_phx4/mp_phx4(3))*(u[4] - u[5]) + (u[14]*hA_p_phx4(3)/mcp_p_phx4(3))*(u[8] - u[5]) + u(17)*P*mp_phx4(3)/(m_f_t*mcp_p_phx4(3))
  d(Tp4_phx4)/dt : Fcn  Expr=(u[13]*Wp_phx4/mp_phx4(4))*(u[5] - u[6]) + (u[14]*hA_p_phx4(4)/mcp_p_phx4(4))*(u[8] - u[5]) + u(17)*P*mp_phx4(4)/(m_f_t*mcp_p_phx4(4))
  d(Ts1_phx4)/dt : Fcn  Expr=(u[15]*Ws_phx4/ms_phx4(1))*(u[2] - u[9]) + (u[16]*hA_s_phx4(1)/mcp_s_phx4(1))*(u[8] - u[9])
  d(Ts2_phx4)/dt : Fcn  Expr=(u[15]*Ws_phx4/ms_phx4(2))*(u[9] - u[10]) + (u[16]*hA_s_phx4(2)/mcp_s_phx4(2))*(u[8] - u[9])
  d(Ts3_phx4)/dt : Fcn  Expr=(u[15]*Ws_phx4/ms_phx4(3))*(u[10] - u[11]) + (u[16]*hA_s_phx4(3)/mcp_s_phx4(3))*(u[7] - u[11])
  d(Ts4_phx4)/dt : Fcn  Expr=(u[15]*Ws_phx4/ms_phx4(4))*(u[11] - u[12]) + (u[16]*hA_s_phx4(4)/mcp_s_phx4(4))*(u[7] - u[11])
  d(Tt1_phx4)/dt : Fcn  Expr=(u[14]*(hA_p_phx4(1) + hA_p_phx4(2))/mcp_t_phx4(1))*(u[3] - u[7]) + (u[16]*(hA_s_phx4(1) + hA_s_phx4(2))/mcp_t_phx4(1))*(u[11] - u[7])
  d(Tt2_phx4)/dt : Fcn  Expr=(u[14]*(hA_p_phx4(3) + hA_p_phx4(4))/mcp_t_phx4(2))*(u[5] - u[8]) + (u[16]*(hA_s_phx4(3) + hA_s_phx4(4))/mcp_t_phx4(2))*(u[9] - u[8])
  PHX4 TEMPERATURES : Outport
  wires:
  Ts1_phx4/1 -> Mux/9
  Ts2_phx4/1 -> Mux/10
  d(Ts2_phx4)/dt/1 -> Ts2_phx4/1
  d(Tp4_phx4)/dt/1 -> Tp4_phx4/1
  Tt1_phx4/1 -> Mux/7
  d(Tp2_phx4)/dt/1 -> Tp2_phx4/1
  Tp4_phx4/1 -> Mux/6
  d(Tt2_phx4)/dt/1 -> Tt2_phx4/1
  SECONDARY FLUID INLET TEMPERATURE/1 -> Mux/2
  Tt2_phx4/1 -> Mux/8
  Mux/1 -> To Workspace/1, PHX4 TEMPERATURES/1, d(Ts4_phx4)/dt/1, d(Ts3_phx4)/dt/1, d(Ts1_phx4)/dt/1, d(Tt2_phx4)/dt/1, d(Tt1_phx4)/dt/1, d(Tp4_phx4)/dt/1, d(Tp3_phx4)/dt/1, d(Tp2_phx4)/dt/1, d(Tp1_phx4)/dt/1, d(Ts2_phx4)/dt/1
  d(Tp1_phx4)/dt/1 -> Tp1_phx4/1
  d(Ts4_phx4)/dt/1 -> Ts4_phx4/1
  Tp1_phx4/1 -> Mux/3
  d(Ts1_phx4)/dt/1 -> Ts1_phx4/1
  d(Ts3_phx4)/dt/1 -> Ts3_phx4/1
  Ts3_phx4/1 -> Mux/11
  Ts4_phx4/1 -> Mux/12
  "Tp3_phx4 "/1 -> Mux/5
  d(Tp3_phx4)/dt/1 -> "Tp3_phx4 "/1
  Tp2_phx4/1 -> Mux/4
  d(Tt1_phx4)/dt/1 -> Tt1_phx4/1
  PRIMARY FLUID INLET TEMPERATURE/1 -> Mux/1
  PRIMARY FLOW FRACTION/1 -> Mux/13
  PRIMARY HEAT TRANSFER FRACTION/1 -> Mux/14
  SECONDARY FLOW FRACTION/1 -> Mux/15
  SECONDARY HEAT TRANSFER FRACTION/1 -> Mux/16
  DECAY HEAT/1 -> Mux/17

== system MSDR_DH_DeplV1sim/HEAT EXCHANGERS/HEAT EXCHANGER LOOP 2/SHX PRIM MIXING ==
  Tp_shx3 : Inport
  Tp_shx4 : Inport  Port=2
  p_flow_frac : Inport  Port=3
  Fcn : Fcn  Expr=u[3]*Wp_shx3/mp_shxm*(u[1]-u[4]) + u[3]*Wp_shx4/mp_shxm*(u[2]-u[4])
  Integrator : Integrator  InitialCondition=T0_p_shx1(4)
  Mux : Mux
  Tp_shx_mix : Outport
  wires:
  Tp_shx3/1 -> Mux/1
  Tp_shx4/1 -> Mux/2
  Mux/1 -> Fcn/1
  p_flow_frac/1 -> Mux/3
  Fcn/1 -> Integrator/1
  Integrator/1 -> Tp_shx_mix/1, Mux/4

== system MSDR_DH_DeplV1sim/HEAT EXCHANGERS/HEAT EXCHANGER LOOP 2/SHX SEC MIXING ==
  Ts_shx3 : Inport
  Ts_shx4 : Inport  Port=2
  s_flow_frac : Inport  Port=3
  Fcn : Fcn  Expr=u[3]*Ws_shx3/ms_shxm*(u[1]-u[4]) + u[3]*Ws_shx4/ms_shxm*(u[2]-u[4])
  Integrator : Integrator  InitialCondition=T0_s_shx1(4)
  Mux : Mux
  Ts_shx_mix : Outport
  wires:
  Ts_shx3/1 -> Mux/1
  Ts_shx4/1 -> Mux/2
  Mux/1 -> Fcn/1
  s_flow_frac/1 -> Mux/3
  Fcn/1 -> Integrator/1
  Integrator/1 -> Ts_shx_mix/1, Mux/4

== system MSDR_DH_DeplV1sim/HEAT EXCHANGERS/HEAT EXCHANGER LOOP 2/SHX//THX PUMP ==
  Clock1 : Clock
  Fcn1 : Fcn  Expr=(1-therm_conv)*exp(-K_pump*(u))+therm_conv
  H.T.C. as f(flow_fraction) : Fcn  Expr=0.8215*u^6-4.108*u^5+7.848*u^4-7.165*u^3+3.004*u^2+0.5903*u+0.008537
  Pump Trip Time : TransportDelay  DelayTime=Trip_T2_pump  BufferSize=4096
  FLOW FRACTION : Outport
  HEAT TRANSFER FRACTION : Outport  Port=2
  wires:
  H.T.C. as f(flow_fraction)/1 -> HEAT TRANSFER FRACTION/1
  Clock1/1 -> Pump Trip Time/1
  Pump Trip Time/1 -> Fcn1/1
  Fcn1/1 -> FLOW FRACTION/1, H.T.C. as f(flow_fraction)/1

== system MSDR_DH_DeplV1sim/HEAT EXCHANGERS/HEAT EXCHANGER LOOP 2/SHX3 HEAT TRANSFER ==
  PRIMARY FLUID INLET TEMPERATURE : Inport
  SECONDARY FLUID INLET TEMPERATURE : Inport  Port=2
  PRIMARY FLOW FRACTION : Inport  Port=3
  PRIMARY HEAT TRANSFER FRACTION : Inport  Port=4
  SECONDARY FLOW FRACTION : Inport  Port=5
  SECONDARY HEAT TRANSFER FRACTION : Inport  Port=6
  Mux : Mux  Inputs=16
      settings: DisplayOption=signals
  To Workspace : ToWorkspace  VariableName=shx3_ht  SampleTime=-1
  Tp1_shx3 : Integrator  InitialCondition=T0_p_shx3(1)
  Tp2_shx3 : Integrator  InitialCondition=T0_p_shx3(2)
  "Tp3_shx3 " : Integrator  InitialCondition=T0_p_shx3(3)
  Tp4_shx3 : Integrator  InitialCondition=T0_p_shx3(4)
  Ts1_shx3 : Integrator  InitialCondition=T0_s_shx3(1)
  Ts2_shx3 : Integrator  InitialCondition=T0_s_shx3(2)
  Ts3_shx3 : Integrator  InitialCondition=T0_s_shx3(3)
  Ts4_shx3 : Integrator  InitialCondition=T0_s_shx3(4)
  Tt1_shx3 : Integrator  InitialCondition=T0_t_shx3(1)
  Tt2_shx3 : Integrator  InitialCondition=T0_t_shx3(2)
  d(Tp1_shx3)/dt : Fcn  Expr=(u[13]*Wp_shx3/mp_shx3(1))*(u[1] - u[3]) + (u[14]*hA_p_shx3(1)/mcp_p_shx3(1))*(u[7] - u[3])
  d(Tp2_shx3)/dt : Fcn  Expr=(u[13]*Wp_shx3/mp_shx3(2))*(u[3] - u[4]) + (u[14]*hA_p_shx3(2)/mcp_p_shx3(2))*(u[7] - u[3])
  d(Tp3_shx3)/dt : Fcn  Expr=(u[13]*Wp_shx3/mp_shx3(3))*(u[4] - u[5]) + (u[14]*hA_p_shx3(3)/mcp_p_shx3(3))*(u[8] - u[5])
  d(Tp4_shx3)/dt : Fcn  Expr=(u[13]*Wp_shx3/mp_shx3(4))*(u[5] - u[6]) + (u[14]*hA_p_shx3(4)/mcp_p_shx3(4))*(u[8] - u[5])
  d(Ts1_shx3)/dt : Fcn  Expr=(u[15]*Ws_shx3/ms_shx3(1))*(u[2] - u[9]) + (u[16]*hA_s_shx3(1)/mcp_s_shx3(1))*(u[8] - u[9])
  d(Ts2_shx3)/dt : Fcn  Expr=(u[15]*Ws_shx3/ms_shx3(2))*(u[9] - u[10]) + (u[16]*hA_s_shx3(2)/mcp_s_shx3(2))*(u[8] - u[9])
  d(Ts3_shx3)/dt : Fcn  Expr=(u[15]*Ws_shx3/ms_shx3(3))*(u[10] - u[11]) + (u[16]*hA_s_shx3(3)/mcp_s_shx3(3))*(u[7] - u[11])
  d(Ts4_shx3)/dt : Fcn  Expr=(u[15]*Ws_shx3/ms_shx3(4))*(u[11] - u[12]) + (u[16]*hA_s_shx3(4)/mcp_s_shx3(4))*(u[7] - u[11])
  d(Tt1_shx3)/dt : Fcn  Expr=(u[14]*(hA_p_shx3(1) + hA_p_shx3(2))/mcp_t_shx3(1))*(u[3] - u[7]) + (u[16]*(hA_s_shx3(1) + hA_s_shx3(2))/mcp_t_shx3(1))*(u[11] - u[7])
  d(Tt2_shx3)/dt : Fcn  Expr=(u[14]*(hA_p_shx4(3) + hA_p_shx4(4))/mcp_t_shx4(2))*(u[5] - u[8]) + (u[16]*(hA_s_shx4(3) + hA_s_shx4(4))/mcp_t_shx4(2))*(u[9] - u[8])
  SHX3 TEMPERATURES : Outport
  wires:
  Ts1_shx3/1 -> Mux/9
  Ts2_shx3/1 -> Mux/10
  d(Ts2_shx3)/dt/1 -> Ts2_shx3/1
  d(Tp4_shx3)/dt/1 -> Tp4_shx3/1
  Tt1_shx3/1 -> Mux/7
  d(Tp2_shx3)/dt/1 -> Tp2_shx3/1
  Tp4_shx3/1 -> Mux/6
  d(Tt2_shx3)/dt/1 -> Tt2_shx3/1
  SECONDARY FLUID INLET TEMPERATURE/1 -> Mux/2
  Tt2_shx3/1 -> Mux/8
  Mux/1 -> To Workspace/1, SHX3 TEMPERATURES/1, d(Ts4_shx3)/dt/1, d(Ts3_shx3)/dt/1, d(Ts2_shx3)/dt/1, d(Ts1_shx3)/dt/1, d(Tt2_shx3)/dt/1, d(Tt1_shx3)/dt/1, d(Tp4_shx3)/dt/1, d(Tp3_shx3)/dt/1, d(Tp2_shx3)/dt/1, d(Tp1_shx3)/dt/1
  d(Tp1_shx3)/dt/1 -> Tp1_shx3/1
  d(Ts4_shx3)/dt/1 -> Ts4_shx3/1
  Tp1_shx3/1 -> Mux/3
  d(Ts1_shx3)/dt/1 -> Ts1_shx3/1
  d(Ts3_shx3)/dt/1 -> Ts3_shx3/1
  Ts3_shx3/1 -> Mux/11
  Ts4_shx3/1 -> Mux/12
  "Tp3_shx3 "/1 -> Mux/5
  d(Tp3_shx3)/dt/1 -> "Tp3_shx3 "/1
  Tp2_shx3/1 -> Mux/4
  d(Tt1_shx3)/dt/1 -> Tt1_shx3/1
  PRIMARY FLUID INLET TEMPERATURE/1 -> Mux/1
  PRIMARY FLOW FRACTION/1 -> Mux/13
  PRIMARY HEAT TRANSFER FRACTION/1 -> Mux/14
  SECONDARY FLOW FRACTION/1 -> Mux/15
  SECONDARY HEAT TRANSFER FRACTION/1 -> Mux/16

== system MSDR_DH_DeplV1sim/HEAT EXCHANGERS/HEAT EXCHANGER LOOP 2/SHX4 HEAT TRANSFER ==
  PRIMARY FLUID INLET TEMPERATURE : Inport
  SECONDARY FLUID INLET TEMPERATURE : Inport  Port=2
  PRIMARY FLOW FRACTION : Inport  Port=3
  PRIMARY HEAT TRANSFER FRACTION : Inport  Port=4
  SECONDARY FLOW FRACTION : Inport  Port=5
  SECONDARY HEAT TRANSFER FRACTION : Inport  Port=6
  Mux : Mux  Inputs=16
      settings: DisplayOption=signals
  To Workspace : ToWorkspace  VariableName=shx4_ht  SampleTime=-1
  Tp1_shx4 : Integrator  InitialCondition=T0_p_shx4(1)
  Tp2_shx4 : Integrator  InitialCondition=T0_p_shx4(2)
  "Tp3_shx4 " : Integrator  InitialCondition=T0_p_shx4(3)
  Tp4_shx4 : Integrator  InitialCondition=T0_p_shx4(4)
  Ts1_shx4 : Integrator  InitialCondition=T0_s_shx4(1)
  Ts2_shx4 : Integrator  InitialCondition=T0_s_shx4(2)
  Ts3_shx4 : Integrator  InitialCondition=T0_s_shx4(3)
  Ts4_shx4 : Integrator  InitialCondition=T0_s_shx4(4)
  Tt1_shx4 : Integrator  InitialCondition=T0_t_shx4(1)
  Tt2_shx4 : Integrator  InitialCondition=T0_t_shx4(2)
  d(Tp1_shx4)/dt : Fcn  Expr=(u[13]*Wp_shx4/mp_shx4(1))*(u[1] - u[3]) + (u[14]*hA_p_shx4(1)/mcp_p_shx4(1))*(u[7] - u[3])
  d(Tp2_shx4)/dt : Fcn  Expr=(u[13]*Wp_shx4/mp_shx4(2))*(u[3] - u[4]) + (u[14]*hA_p_shx4(2)/mcp_p_shx4(2))*(u[7] - u[3])
  d(Tp3_shx4)/dt : Fcn  Expr=(u[13]*Wp_shx4/mp_shx4(3))*(u[4] - u[5]) + (u[14]*hA_p_shx4(3)/mcp_p_shx4(3))*(u[8] - u[5])
  d(Tp4_shx4)/dt : Fcn  Expr=(u[13]*Wp_shx4/mp_shx4(4))*(u[5] - u[6]) + (u[14]*hA_p_shx4(4)/mcp_p_shx4(4))*(u[8] - u[5])
  d(Ts1_shx4)/dt : Fcn  Expr=(u[15]*Ws_shx4/ms_shx4(1))*(u[2] - u[9]) + (u[16]*hA_s_shx4(1)/mcp_s_shx4(1))*(u[8] - u[9])
  d(Ts2_shx4)/dt : Fcn  Expr=(u[15]*Ws_shx4/ms_shx4(2))*(u[9] - u[10]) + (u[16]*hA_s_shx4(2)/mcp_s_shx4(2))*(u[8] - u[9])
  d(Ts3_shx4)/dt : Fcn  Expr=(u[15]*Ws_shx4/ms_shx4(3))*(u[10] - u[11]) + (u[16]*hA_s_shx4(3)/mcp_s_shx4(3))*(u[7] - u[11])
  d(Ts4_shx4)/dt : Fcn  Expr=(u[15]*Ws_shx4/ms_shx4(4))*(u[11] - u[12]) + (u[16]*hA_s_shx4(4)/mcp_s_shx4(4))*(u[7] - u[11])
  d(Tt1_shx4)/dt : Fcn  Expr=(u[14]*(hA_p_shx4(1) + hA_p_shx4(2))/mcp_t_shx4(1))*(u[3] - u[7]) + (u[16]*(hA_s_shx4(1) + hA_s_shx4(2))/mcp_t_shx4(1))*(u[11] - u[7])
  d(Tt2_shx4)/dt : Fcn  Expr=(u[14]*(hA_p_shx4(3) + hA_p_shx4(4))/mcp_t_shx4(2))*(u[5] - u[8]) + (u[16]*(hA_s_shx4(3) + hA_s_shx4(4))/mcp_t_shx4(2))*(u[9] - u[8])
  SHX4 TEMPERATURES : Outport
  wires:
  Ts1_shx4/1 -> Mux/9
  Ts2_shx4/1 -> Mux/10
  d(Ts2_shx4)/dt/1 -> Ts2_shx4/1
  d(Tp4_shx4)/dt/1 -> Tp4_shx4/1
  Tt1_shx4/1 -> Mux/7
  d(Tp2_shx4)/dt/1 -> Tp2_shx4/1
  Tp4_shx4/1 -> Mux/6
  d(Tt2_shx4)/dt/1 -> Tt2_shx4/1
  SECONDARY FLUID INLET TEMPERATURE/1 -> Mux/2
  Tt2_shx4/1 -> Mux/8
  Mux/1 -> To Workspace/1, SHX4 TEMPERATURES/1, d(Ts4_shx4)/dt/1, d(Ts3_shx4)/dt/1, d(Ts2_shx4)/dt/1, d(Ts1_shx4)/dt/1, d(Tt2_shx4)/dt/1, d(Tt1_shx4)/dt/1, d(Tp4_shx4)/dt/1, d(Tp3_shx4)/dt/1, d(Tp2_shx4)/dt/1, d(Tp1_shx4)/dt/1
  d(Tp1_shx4)/dt/1 -> Tp1_shx4/1
  d(Ts4_shx4)/dt/1 -> Ts4_shx4/1
  Tp1_shx4/1 -> Mux/3
  d(Ts1_shx4)/dt/1 -> Ts1_shx4/1
  d(Ts3_shx4)/dt/1 -> Ts3_shx4/1
  Ts3_shx4/1 -> Mux/11
  Ts4_shx4/1 -> Mux/12
  "Tp3_shx4 "/1 -> Mux/5
  d(Tp3_shx4)/dt/1 -> "Tp3_shx4 "/1
  Tp2_shx4/1 -> Mux/4
  d(Tt1_shx4)/dt/1 -> Tt1_shx4/1
  PRIMARY FLUID INLET TEMPERATURE/1 -> Mux/1
  PRIMARY FLOW FRACTION/1 -> Mux/13
  PRIMARY HEAT TRANSFER FRACTION/1 -> Mux/14
  SECONDARY FLOW FRACTION/1 -> Mux/15
  SECONDARY HEAT TRANSFER FRACTION/1 -> Mux/16

== system MSDR_DH_DeplV1sim/HEAT EXCHANGERS/HEAT EXCHANGER LOOP 3/PHX PRIM MIXING ==
  Tp_phx5 : Inport
  Tp_phx6 : Inport  Port=2
  p_flow_frac : Inport  Port=3
  Decay Heat : Inport  Port=4
  Fcn : Fcn  Expr="u[3]*Wp_phx5/mp_phxm*(u[1]-u[4]) + u[3]*Wp_phx6/mp_phxm*(u[2]-u[4])  + u(5)*P*mp_phxm/(m_f_t*mp_phxm*Cp_f)"
  Integrator : Integrator  InitialCondition=Tf_in
  Mux : Mux  Inputs=5
  Tp_phx_mix : Outport
  wires:
  Tp_phx5/1 -> Mux/1
  Tp_phx6/1 -> Mux/2
  Mux/1 -> Fcn/1
  p_flow_frac/1 -> Mux/3
  Fcn/1 -> Integrator/1
  Integrator/1 -> Tp_phx_mix/1, Mux/4
  Decay Heat/1 -> Mux/5

== system MSDR_DH_DeplV1sim/HEAT EXCHANGERS/HEAT EXCHANGER LOOP 3/PHX SEC MIXING ==
  Ts_phx5 : Inport
  Ts_phx6 : Inport  Port=2
  s_flow_frac : Inport  Port=3
  Fcn : Fcn  Expr=u[3]*Ws_phx5/ms_phxm*(u[1]-u[4]) + u[3]*Ws_phx6/ms_phxm*(u[2]-u[4])
  Integrator : Integrator  InitialCondition=T0_s_phx1(4)
  Mux : Mux
  Ts_phx_mix : Outport
  wires:
  Ts_phx5/1 -> Mux/1
  Ts_phx6/1 -> Mux/2
  Mux/1 -> Fcn/1
  s_flow_frac/1 -> Mux/3
  Fcn/1 -> Integrator/1
  Integrator/1 -> Ts_phx_mix/1, Mux/4

== system MSDR_DH_DeplV1sim/HEAT EXCHANGERS/HEAT EXCHANGER LOOP 3/PHX//SHX PUMP ==
  Clock1 : Clock
  Fcn1 : Fcn  Expr=(1-therm_conv)*exp(-K_pump*(u))+therm_conv
  H.T.C. as f(flow_fraction) : Fcn  Expr=0.8215*u^6-4.108*u^5+7.848*u^4-7.165*u^3+3.004*u^2+0.5903*u+0.008537
  Pump Trip Time : TransportDelay  DelayTime=Trip_S3_pump  BufferSize=4096
  FLOW FRACTION : Outport
  HEAT TRANSFER FRACTION : Outport  Port=2
  wires:
  H.T.C. as f(flow_fraction)/1 -> HEAT TRANSFER FRACTION/1
  Clock1/1 -> Pump Trip Time/1
  Pump Trip Time/1 -> Fcn1/1
  Fcn1/1 -> FLOW FRACTION/1, H.T.C. as f(flow_fraction)/1
